simulink model "sl_ctorque"  (R2019b)
settings: Solver=ode23t  StartTime=0.0  StopTime=10  FixedStep=0.01  MaxStep=0.05  RelTol=1e-3  EnableMultiTasking=on
PreLoadFcn:
  | mdl_puma560
values from neighbouring files (symbols this model uses):
  q = jtraj(POS(1,:), POS(4,:), 10)    [Model_210F.m]    (also in Model_210F_old.m; ThreeMilIt_Anim.mat = [1 -0.666666666667 1 1 -0.666666666667 -0.666666666667 1 -0.; WorkspContrPointToPoint.mat = [0 1.3110137073e-12 5.24405294824e-12 1.17991149051e-11 2.09; matlab.mat = [0 1.3110137073e-12 5.24405294824e-12 1.17991149051e-11 2.09)
  qd = [0 4.76434506416e-07 9.52868500387e-07 1.4293019828e-06 1.90573495456e-06 4.2878921846e-06 6.67003678183e-06 9.0521688577e-06 1.14342885237e-05 2.33447046064e-05 3.52548271627e-05 4.71646701285e-05 ... (62478 elements, 10413x6)]    [WorkspContrPointToPoint.mat]    (also in matlab.mat)
  qdd = [0 -0.228939437467 -0.422657423016 -0.583007717274 -0.711844080869 -0.811020274427 -0.882390058577 -0.927807193945 -0.949125441158 -0.948198560844 -0.926880313631 -0.887024460145 ... (246 elements, 41x6)]    [WorkspContrPointToPoint.mat]    (also in matlab.mat = [0 -0.36798417892 -0.679355407237 -0.93709331393 -1.14417752)
  R = SerialLink(L, 'name', '210F', 'comment', 'six DOF', 'manufacturer', 'FANUC')    [Model_210F.m]    (also in Model_210F_old.m)
undefined symbols (not defined in the file or in its folder): slcoulomb
libraries: roblocks x15, simulink x1
settings Model: ExtModeTrigMode=oneshot  ExtModeArmWhenConnect=off  Creator=pic  LastModifiedBy=Karl
settings SolverCC: ZeroCrossControl=DisableAll
settings DataIOCC: SaveFormat=Array  SignalLoggingSaveFormat=ModelDataLogs  TimeSaveName=t  OutputSaveName=y  ReturnWorkspaceOutputsName=ctorque
settings OptimizationCC: BlockReduction=off  BooleanDataType=off  ExpressionDepthLimit=2147483647  InitFltsAndDblsToZero=on  LifeSpan=inf
settings DebuggingCC: SaveWithParameterizedLinksMsg=none  UnderspecifiedInitializationDetection=Classic  MergeDetectMultiDrivingBlocksExec=none  SignalResolutionControl=TryResolveAllWithWarning  MultiTaskDSMMsg=warning  MultiTaskCondExecSysMsg=none  FcnCallInpInsideContextMsg=warning  AllowSymbolicDim=off  StateNameClashWarn=warning  SFUnexpectedBacktrackingDiag=warning  SFNoUnconditionalDefaultTransitionDiag=warning  SFExecutionAtInitializationDiag=none  ArithmeticOperatorsInVariantConditions=warning
settings HardwareCC: ProdBitPerPointer=32  ProdBitPerSizeT=32  ProdBitPerPtrDiffT=32  ProdLargestAtomicFloat=None  ProdIntDivRoundTo=Undefined  ProdEndianess=Unspecified  ProdWordSize=32  ProdHWDeviceType=32-bit Generic  TargetUnknown=on
settings ModelReferenceCC: PropagateSignalLabelsOutOfModel=off
settings SFSimCC: SimUseLocalCustomCode=off  CustomCodeUndefinedFunction=UseInterfaceOnly
settings RTWCC: RTWUseLocalCustomCode=off
settings CodeAppCC: StateflowObjectComments=on
settings GRTTargetCC: TargetLangStandard=C89/C90 (ANSI)  ModelReferenceCompliant=off  CompOptLevelCompliant=off  GeneratePreprocessorConditionals=Disable all  CombineOutputUpdateFcns=off  MatFileLogging=off  GRTInterface=on
settings ConfigComp: CovMetricSettings=dw  CovHtmlReporting=on  CovSaveCumulativeToWorkspaceVar=on  CovSaveSingleToWorkspaceVar=on  CovExternalEMLEnable=off

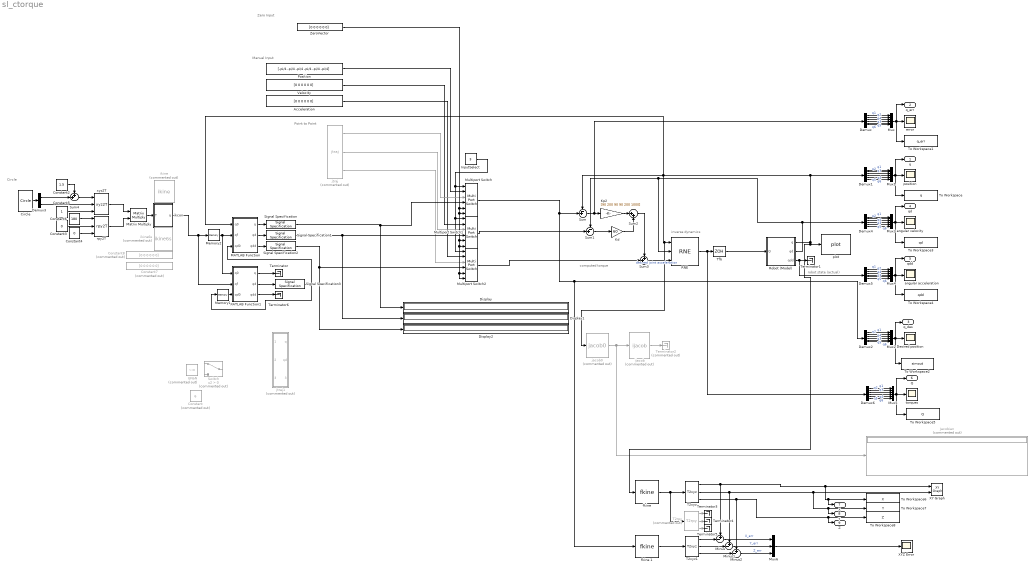
== system sl_ctorque ==
  note: Circle
  note: Point to Point
  note: Manual Input
  note: Zero Input
  note: inverse dynamics
  note: computed torque
  note: robot state
      | (actual)
  Acceleration : Constant  Value=[0 0 0 0 0 0]
  Circle : roblocks/Toolbox/Circle  radius=0.5  freq=0.1
  Constant : Constant  Commented=on  Value=6
  Constant2 : Constant  Value=1.5
  Constant3 : Constant  Value=0
  Constant4 : Constant  Value=0
  Constant5 : Constant
  Constant6 : Constant  Value=180
  Constant7 : Constant  Commented=on  Value=[0 0 0 0 0 0]
  Constant8 : Constant  Commented=on  Value=[0 0 0 0 0 0]
  Demux{,1..2,4..6} (6 alike) : Demux  Outputs=6
  Demux3 : Demux  Outputs=2
  Desired position : Scope
  Display : Display
  Display1 : Display
  Display2 : Display
  InputSelect : Constant  Value=3
  IsNaN : RelationalOperator  Commented=on  Operator=~=  OutDataTypeStr=boolean  RndMeth=Simplest
  Jacobian : Display  Commented=on
  Kd : Gain  Gain=60  SaturateOnIntegerOverflow=on  OutDataTypeStr=Inherit: Same as input  ParamDataTypeStr=Inherit: Same as input
  Kp2 : Gain  Gain=[90 200 90 90 200 1000]  SaturateOnIntegerOverflow=on  OutDataTypeStr=Inherit: Same as input  ParamDataTypeStr=Inherit: Same as input
  MATLAB Function : MATLAB Function  TreatAsAtomicUnit=on
  MATLAB Function1 : MATLAB Function  TreatAsAtomicUnit=on
  Matrix Multiply : Product  Multiplication=Matrix(*)
  Memory1 : Memory  InitialCondition=[0 0 0 0 0 0]  InheritSampleTime=on
  Memory2 : Memory  InitialCondition=[0 0 0 0 0 0]  InheritSampleTime=on
  Minus : Sum  Inputs=+-|
  Minus1 : Sum  Inputs=+-|
  Minus2 : Sum  Inputs=+-|
  Multiport Switch : MultiPortSwitch  Inputs=5
  Multiport Switch1 : MultiPortSwitch  Inputs=5
  Multiport Switch2 : MultiPortSwitch  Inputs=5
  Mux{,1..5} (6 alike) : Mux  Inputs=6
  Mux6 : Mux  Inputs=3
  Position : Constant  Value=[-pi/4 -pi/4 -pi/4 -pi/4 -pi/4 -pi/4]
  RNE : roblocks/Arm/RNE  robot=R.nofriction  grav=[0 0 9.81]
  Robot (Model) : Subsystem  AncestorBlock=roblocks/Arm/Robot  mask{robot=R.nofriction, q0=[0 -pi/4 0 0 -pi/4 0]}
      mask prompts: robot "Robot object"; q0 "Initial state"
      mask help: Rigid-body dynamic model of robot.
      mask init:
      | if isa(robot, 'SerialLink')
      |     rname = robot.name;
      |     %fprintf('**robot name is %s\n', rname);
      | else
      |     rname = '';
      |     n = 0
      | end
      mask Help:
      | Simulates the forward (direct) rigid-body dynamics of the robot described
      | by the given robot object.  For given applied joint torque/force it computes
      | the instaneous joint coordinates, velocities and acclerations.
      | 
      | 
      | <b>Parameters::</b>
      | 
      | robot (SerialLink) a dynamic model of an N-link serial link manipulator
      | q0 (1xN)  Initial joint coordinates
      | 
      | <b>Inputs::</b>
      | 
      | Q (1xN) the generalized joint force (torque or force) required to achieve
      | the motion state (q, qd, qdd).
      | 
      | <b>Outputs::</b>
      | 
      | q (1xN) joint coordinates
      | qd (1xN) joint coordinate velocity
      | qdd (1xN) joint coordinate acceleration
      | 
      | 
      | <b>Notes::</b>
      | 
      | - Required to simulate robot rigid body motion.
      | - Implemented using the recursive Newton-Euler scheme (RNE).
      | - A wrapper for the Toolbox method accel() which in turn depends on the
      |   method rne().
      mask Display:
      | port_label('input', 1, 'Q')
      | port_label('output', 1, 'q')
      | port_label('output', 2, 'qd')
      | port_label('output', 3, 'qdd')
      | text(0.1, 0.9,  rname, 'horizontalAlignment', 'left')
  Signal Specification{,1..3} (4 alike) : SignalSpecification  Dimensions=6
  Sum : Sum  Inputs=-+|  SaturateOnIntegerOverflow=on  InputSameDT=on  OutDataTypeStr=Inherit: Same as first input
  Sum1 : Sum  Inputs=-+|  SaturateOnIntegerOverflow=on  InputSameDT=on  OutDataTypeStr=Inherit: Same as first input
  Sum2 : Sum  Inputs=|++  SaturateOnIntegerOverflow=on  InputSameDT=on  OutDataTypeStr=Inherit: Same as first input
  Sum3 : Sum  Inputs=++|  SaturateOnIntegerOverflow=on  InputSameDT=on  OutDataTypeStr=Inherit: Same as first input
  Sum4 : Sum  Inputs=++|
  Switch : Switch  Commented=on  Criteria=u2 > Threshold
  T2rpy : roblocks/Toolbox/T2rpy  Commented=on  sequence=ZYX  degrees=off
  T2xyz : roblocks/Toolbox/T2xyz
  T2xyz1 : roblocks/Toolbox/T2xyz
  Terminator{,1,3..6} (6 alike) : Terminator
  Terminator2 : Terminator  Commented=on
  Tfb : ZeroOrderHold  SampleTime=0.005
  To Workspace : ToWorkspace  VariableName=q  SaveFormat=Timeseries  SampleTime=-1
  To Workspace1 : ToWorkspace  VariableName=q_err  SaveFormat=Timeseries  SampleTime=-1
  To Workspace2 : ToWorkspace  VariableName=simout  SaveFormat=Timeseries  SampleTime=-1
  To Workspace3 : ToWorkspace  VariableName=qd  SaveFormat=Timeseries  SampleTime=-1
  To Workspace4 : ToWorkspace  VariableName=qdd  SaveFormat=Timeseries  SampleTime=-1
  To Workspace5 : ToWorkspace  VariableName=Q  SaveFormat=Timeseries  SampleTime=-1
  To Workspace6 : ToWorkspace  VariableName=X  SaveFormat=Timeseries  SampleTime=-1
  To Workspace7 : ToWorkspace  VariableName=Y  SaveFormat=Timeseries  SampleTime=-1
  To Workspace8 : ToWorkspace  VariableName=Z  SaveFormat=Timeseries  SampleTime=-1
  Velocity : Constant  Value=[0 0 0 0 0 0]
  XY Graph : simulink/Sinks/XY Graph  xmin=-3  xmax=3  ymin=-3  ymax=3  st=-1
  XYZ Error : Scope
  ZeroVector : Constant  Value=[0 0 0 0 0 0]
  angular acceleration : Scope
  angular velocity : Scope
  error : Scope
  "fkine " : roblocks/Arm/fkine  robot=R.nofriction
  fkine 1 : roblocks/Arm/fkine  robot=R.nofriction
  "ijacob " : roblocks/Arm/ijacob  Commented=on
  ikcon : Subsystem  mask{robot=R}
      mask prompts: robot "Robot object"
      mask help: Inverse kinematics for 6-axis spherical robot
      mask Help:
      | Compute joint coordinates for robot given end-effector pose.
      | 
      | 
      | <b>Parameters::</b>
      | 
      | Robot (SerialLink class)  The N-axis robot object for computing forward kinematics.
      | Configuration             Configuration string comprised of 'lrudnf'
      | 
      | <b>Inputs::</b>
      | 
      | T (4x4) the pose of the end effector as a homogeneous transformation
      | 
      | 
      | <b>Outputs::</b>
      | 
      | q (1xN) joint coordinates
      | 
      | <b>Notes::</b>
      | 
      | - A wrapper for the Toolbox method ikine6s().
  ikine : roblocks/Arm/ikine  Commented=on  robot=R.nofriction  q0=[0 -pi/4 0 0 -pi/4 0]  M=[1 1 1 1 1 1]  pinv=off  options={}
  ikine6s : roblocks/Arm/ikine6s  Commented=on  robot=R  conf='luf'
  "jacob0 " : roblocks/Arm/jacob0   Commented=on  robot=R
  jtraj : roblocks/Toolbox/jtraj  Commented=on  q0=[0 0 0 0 0 0]  qf=[-pi/4 -pi/4 -pi/4 -pi/4 -pi/4 -pi/4]  tmax=5  ts=-1
  jtraj1 : Subsystem  Commented=on  mask{q0=[0 0 0 0 0 0], qf=[-pi/4 -pi/4 -pi/4 -pi/4 -pi/4 -pi/4], tmax=5, ts=-1}
      mask prompts: tmax "tmax (s)"; ts "ts (s)"
      mask help: Joint interpolated trajectory.
      mask init:
      | n = length(q0);
      | if length(q0) ~= length(qf) ,
      |  error('q0 and qf must be same length')
      | end
      | t=[0:100]'/100*tmax;
      | [q,qd,qdd] = jtraj(q0, qf, t);
      mask Help:
      | Generate quintic polynomial to move from initial to final joint angles as specified.  Initial and final velocity are assumed to be zero.
      | 
      | <b>Parameters::</b>
      | 
      | q0 (1xN) initial joint coordinates
      | qf (1xN) final joint coordinates
      | tmax (1x1) the time for the trajectory to complete
      | 
      | Initial and final velocity are assumed to be zero.
      | 
      | <b>Outputs::</b>
      | 
      | q (1xN) vector of joint coordinates at current simulation time
      | qd (1xN) vector of joint coordinate velocity at current simulation time
      | qdd (1xN) vector of joint coordinate acceleration at current simulation time
      | 
      | <b>Notes::</b>
      | 
      | - If simulation time exceeds tmax then q is clipped to qf.
      | - A wrapper on the Toolbox function jtraj.
      | - The piecewise constant output of jtraj is interpolated to the current
      |   simulation time.
      mask Display:
      | port_label('output', 1, 'q')
      | port_label('output', 2, 'qd')
      | port_label('output', 3, 'qdd')
      | 
      | port_label('input', 1, 'q0')
      | port_label('input', 2, 'qf')
      | port_label('input', 3, 'tmax')
  plot : roblocks/Arm/plot  robot=R.nofriction  fps=10  holdplot=on
  position : Scope
  rpy2T : roblocks/Toolbox/rpy2T  sequence=ZYX  degrees=on
  torques : Scope
  xyz2T : roblocks/Toolbox/xyz2T
  q : Outport  VectorParamsAs1DForOutWhenUnconnected=off
  q_err : Outport  Port=2  VectorParamsAs1DForOutWhenUnconnected=off
  q_des : Outport  Port=3
  qd : Outport  Port=4  VectorParamsAs1DForOutWhenUnconnected=off
  qdd : Outport  Port=5  VectorParamsAs1DForOutWhenUnconnected=off
  Q : Outport  Port=6  VectorParamsAs1DForOutWhenUnconnected=off
  X : Outport  Port=7  VectorParamsAs1DForOutWhenUnconnected=off
  Y : Outport  Port=8  VectorParamsAs1DForOutWhenUnconnected=off
  Z : Outport  Port=9
  wires:
  Kp2/1 -> Sum2/1
  RNE/1 -> Demux6/1, Tfb/1
  Kd/1 -> Sum2/2
  Sum3/1 -> RNE/3  "desired joint acceleration"
  Sum2/1 -> Sum3/1
  Mux/1 -> q_err/1, To Workspace1/1, error/1
  Demux/4 -> Mux/4  "q4"
  Demux/5 -> Mux/5  "q5"
  Demux/6 -> Mux/6  "q6"
  Demux/3 -> Mux/3  "q3"
  Demux/2 -> Mux/2  "q2"
  Sum/1 -> Kp2/1, Demux/1
  Demux/1 -> Mux/1  "q1"
  Mux1/1 -> q/1, To Workspace/1, position/1
  Demux1/6 -> Mux1/6  "q6"
  Demux1/3 -> Mux1/3  "q3"
  Demux1/2 -> Mux1/2  "q2"
  Demux1/5 -> Mux1/5  "q5"
  Demux1/1 -> Mux1/1  "q1"
  Demux1/4 -> Mux1/4  "q4"
  Demux2/4 -> Mux2/4  "q4"
  Multiport Switch/1 -> fkine 1/1, Demux2/1, Sum/2
  Demux2/1 -> Mux2/1  "q1"
  Demux2/5 -> Mux2/5  "q5"
  Demux2/2 -> Mux2/2  "q2"
  Demux2/3 -> Mux2/3  "q3"
  Demux2/6 -> Mux2/6  "q6"
  Mux2/1 -> Desired position/1, q_des/1, To Workspace2/1
  Multiport Switch1/1 -> Sum1/2
  Multiport Switch2/1 -> Sum3/2
  xyz2T/1 -> Matrix Multiply/1
  rpy2T/1 -> Matrix Multiply/2
  Sum4/1 -> xyz2T/1
  Demux3/2 -> xyz2T/2
  Demux3/1 -> Sum4/2
  Constant3/1 -> rpy2T/2
  Circle/1 -> Demux3/1
  Constant6/1 -> rpy2T/1
  Constant2/1 -> Sum4/1
  Constant5/1 -> xyz2T/3
  Matrix Multiply/1 -> ikcon/1(T)
  Robot (Model)/2(qd) -> Demux4/1, Sum1/1, RNE/2
  Demux4/1 -> Mux3/1  "q1"
  Mux3/1 -> qd/1, To Workspace3/1, angular velocity/1
  Demux4/5 -> Mux3/5  "q5"
  Demux4/2 -> Mux3/2  "q2"
  Demux4/6 -> Mux3/6  "q6"
  Demux4/4 -> Mux3/4  "q4"
  Demux4/3 -> Mux3/3  "q3"
  Demux5/2 -> Mux4/2  "q2"
  Demux5/5 -> Mux4/5  "q5"
  Demux5/6 -> Mux4/6  "q6"
  Robot (Model)/3(qdd) -> Demux5/1, Terminator1/1
  Mux4/1 -> qdd/1, To Workspace4/1, angular acceleration/1
  Demux5/1 -> Mux4/1  "q1"
  Demux5/4 -> Mux4/4  "q4"
  Demux5/3 -> Mux4/3  "q3"
  Sum1/1 -> Kd/1
  Demux6/1 -> Mux5/1  "q1"
  Demux6/3 -> Mux5/3  "q3"
  Mux5/1 -> Q/1, To Workspace5/1, torques/1
  Demux6/6 -> Mux5/6  "q6"
  Demux6/2 -> Mux5/2  "q2"
  Demux6/4 -> Mux5/4  "q4"
  Demux6/5 -> Mux5/5  "q5"
  InputSelect/1 -> Multiport Switch/1, Multiport Switch1/1, Multiport Switch2/1
  Position/1 -> Multiport Switch/2
  Velocity/1 -> Multiport Switch1/2
  Acceleration/1 -> Multiport Switch2/2
  jtraj/1 -> Multiport Switch/3
  jtraj/2 -> Multiport Switch1/3
  jtraj/3 -> Multiport Switch2/3
  Signal Specification1/1 -> Display1/1, Multiport Switch1/4
  Signal Specification2/1 -> Multiport Switch2/4, Display2/1
  "jacob0 "/1 -> Jacobian/1, "ijacob "/1
  ZeroVector/1 -> Multiport Switch/5, Multiport Switch/6, Multiport Switch1/5, Multiport Switch1/6, Multiport Switch2/5, Multiport Switch2/6
  Constant4/1 -> rpy2T/3
  "ijacob "/1 -> Terminator2/1
  "fkine "/1 -> T2rpy/1, T2xyz/1
  T2xyz/1 -> Minus/1, X/1, To Workspace6/1, XY Graph/1
  T2xyz/2 -> Minus1/1, To Workspace7/1, Y/1, XY Graph/2
  T2xyz/3 -> To Workspace8/1, Z/1, Minus2/1
  T2rpy/1 -> Terminator3/1
  T2rpy/2 -> Terminator4/1
  T2rpy/3 -> Terminator5/1
  Robot (Model)/1(q) -> "fkine "/1, plot/1, Demux1/1, MATLAB Function/1(q0), Sum/1, "jacob0 "/1, RNE/1
  Signal Specification/1 -> Multiport Switch/4, Display/1
  Tfb/1 -> Robot (Model)/1(Q)
  Memory2/1 -> MATLAB Function/2(qf), MATLAB Function1/1(q0)
  MATLAB Function/1(q) -> Signal Specification/1
  MATLAB Function/2(qd) -> Signal Specification1/1
  MATLAB Function/3(qdd) -> Signal Specification2/1
  fkine 1/1 -> T2xyz1/1
  T2xyz1/1 -> Minus/2
  T2xyz1/2 -> Minus1/2
  T2xyz1/3 -> Minus2/2
  Minus/1 -> Mux6/1  "X_err"
  Minus2/1 -> Mux6/3  "Z_err"
  Minus1/1 -> Mux6/2  "Y_err"
  Mux6/1 -> XYZ Error/1
  ikcon/1(q) -> MATLAB Function1/2(qf), Memory2/1
  Signal Specification3/1 -> Memory1/1, MATLAB Function/3(qd0)
  MATLAB Function1/1(q) -> Terminator/1
  MATLAB Function1/3(qdd) -> Terminator6/1
  Memory1/1 -> MATLAB Function1/3(qd0)
  MATLAB Function1/2(qd) -> Signal Specification3/1

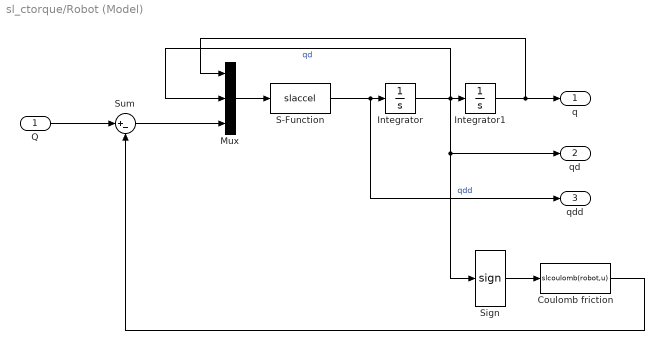
== system sl_ctorque/Robot (Model) ==
  Q : Inport
  Coulomb friction : MATLABFcn  MATLABFcn=slcoulomb(robot,u)  OutputDimensions=[robot.n 1]  Output1D=off
  Integrator : Integrator
  Integrator1 : Integrator  InitialCondition=q0
  Mux : Mux  Inputs=3
  S-Function : S-Function  FunctionName=slaccel  Parameters=robot  SFunctionDeploymentMode=off  EnableBusSupport=off
  Sign : Signum
  Sum : Sum  Inputs=|+-
  q : Outport  VectorParamsAs1DForOutWhenUnconnected=off
  qd : Outport  Port=2  VectorParamsAs1DForOutWhenUnconnected=off
  qdd : Outport  Port=3  VectorParamsAs1DForOutWhenUnconnected=off
  wires:
  S-Function/1 -> qdd/1, Integrator/1  "qdd"
  Mux/1 -> S-Function/1
  Integrator/1 -> Sign/1, qd/1, Integrator1/1, Mux/2  "qd"
  Integrator1/1 -> q/1, Mux/1
  Q/1 -> Sum/1
  Sum/1 -> Mux/3
  Coulomb friction/1 -> Sum/2
  Sign/1 -> Coulomb friction/1

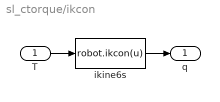
== system sl_ctorque/ikcon ==
  T : Inport
  ikine6s : MATLABFcn  MATLABFcn=robot.ikcon(u)  OutputDimensions=6
  q : Outport  VectorParamsAs1DForOutWhenUnconnected=off
  wires:
  T/1 -> ikine6s/1
  ikine6s/1 -> q/1

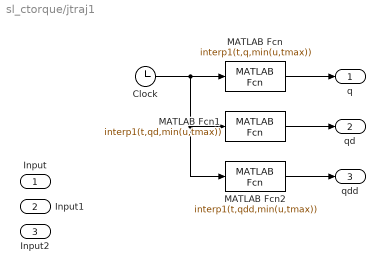
== system sl_ctorque/jtraj1 ==
  Input : Inport
  Input1 : Inport  Port=2
  Input2 : Inport  Port=3
  Clock : Clock
  MATLAB Fcn : MATLABFcn  MATLABFcn=interp1(t,q,min(u,tmax))  OutputDimensions=n  SampleTime=ts
  MATLAB Fcn1 : MATLABFcn  MATLABFcn=interp1(t,qd,min(u,tmax))  OutputDimensions=n  SampleTime=ts
  MATLAB Fcn2 : MATLABFcn  MATLABFcn=interp1(t,qdd,min(u,tmax))  OutputDimensions=n  SampleTime=ts
  q : Outport  VectorParamsAs1DForOutWhenUnconnected=off
  qd : Outport  Port=2  VectorParamsAs1DForOutWhenUnconnected=off
  qdd : Outport  Port=3  VectorParamsAs1DForOutWhenUnconnected=off
  wires:
  MATLAB Fcn2/1 -> qdd/1
  Clock/1 -> MATLAB Fcn2/1, MATLAB Fcn1/1, MATLAB Fcn/1
  MATLAB Fcn1/1 -> qd/1
  MATLAB Fcn/1 -> q/1

== matlab function sl_ctorque/MATLAB Function1 ==
  data: q0 input; q output; qf input; qd output; qdd output; qd0 input
function [q,qd,qdd]= fcn(q0,qf,qd0)
[q_,qd_,qdd_] = jtraj(q0, qf, 2,qd0,qd0);
q=q_(2,:);
qd=qd_(2,:);
qdd=qdd_(2,:);
end

== matlab function sl_ctorque/MATLAB Function ==
  data: q0 input; q output; qf input; qd output; qdd output; qd0 input
function [q,qd,qdd]= fcn(q0,qf,qd0)
[q_,qd_,qdd_] = jtraj(q0, qf, 2,qd0,qd0);
q=q_(2,:);
qd=qd_(2,:);
qdd=qdd_(2,:);
end
